simulink model "VFlexP"  (R2025a)
settings: Solver=ode23tb  StartTime=0.0  StopTime=40  FixedStep=5e-5
model workspace (MAT data in the model file):
  DCop_DCBUCK : object (value not decoded)
  Grid_CCVSC_idx = [2; 3; 4; 5; 6; 7; 8; 9; 10; 11; 12]
  Grid_CCVSCs = 1
  Grid_CCVSCs_buses = 1
  Grid_CCVSCs_toM = [0 1 0 0 0 0 0 0 0 0 0 0 ... (781 elements, 71x11)]
  Grid_C_Lines = [0.1 0.1 0.1 0.1]
  Grid_Cbuses = [0.05000002 0.10000002 0.10000002 0.10000002 0.05000002]
  Grid_DC : object (value not decoded)
  Grid_DCop_DCBUCK : object (value not decoded)
  Grid_DCop_DC_PES : object (value not decoded)
  Grid_DFIGs = 1
  Grid_DFIGs_buses = 1
  Grid_DGs : string (value not decoded)
  Grid_From_buses = [1 2 4 4]
  Grid_GFls = 1
  Grid_GFls_buses = 1
  Grid_GFr_idx = [1; 2; 3]
  Grid_GFrs = 1
  Grid_GFrs_buses = 1
  Grid_GFrs_toM = [1 0 0 0 0 0 0 0 0 1 0 0 ... (15 elements, 5x3)]
  Grid_IG_idx = 1
  Grid_IGs = 1
  Grid_IGs_buses = 1
  Grid_IGs_toM = [1; 0]
  Grid_L_Lines = [0.5 0.5 0.5 0.5]
  Grid_L_Loads = [0.000959999944704 0.000156249997559 0.00154855477548]
  Grid_Lines_fromM : object (value not decoded)
  Grid_Lines_toM : object (value not decoded)
  Grid_Load_buses = [2; 3; 4]
  Grid_Load_busesDC = []
  Grid_MGES_idx = [1; 2; 3]
  Grid_MGESs = 1
  Grid_MGESs_buses = [1; 5; 3]
  Grid_MGESs_toM = [1 0 0 0 0 0 0 0 0 1 0 0 ... (15 elements, 5x3)]
  Grid_MSGs = 1
  Grid_MSGs_buses = 1
  Grid_Nbuses = 5
  Grid_PQ_gen = [3; 2; 2]
  Grid_Ploads = [1250 4000 1250]
  Grid_PloadsDC = []
  Grid_Ps_lf = [0.274439537683 0.78 0.3]
  Grid_Qloads = [0.3 0.5 0.5]
  Grid_Qs_lf = [-0.0366071562958 0.126505596722 -0.0162964024532]
  Grid_R_Lines = [0.01 0.01 0.01 0.01]
  Grid_R_Loads = [3.9999997696 1.24999998047 3.8713869387]
  Grid_R_Loads_DC = 0
  Grid_Rcf = [50000000 50000000 50000000 50000000 50000000]
  Grid_SCs = 1
  Grid_SCs_buses = 1
  Grid_SG_idx = 1
  Grid_SGs = 1
  Grid_SGs_buses = 1
  Grid_SGs_toM = [1; 0]
  Grid_To_buses = [2 3 3 5]
  Grid_VCVSC_idx = [1; 2; 3; 4; 5; 6; 7; 8; 9; 10; 11; 12]
  Grid_VCVSCs = 1
  Grid_VCVSCs_buses = [1; 2; 3; 6; 8; 9; 12; 58; 59; 60; 63; 65]
  Grid_VCVSCs_toM = [1 0 0 0 0 0 0 0 0 0 0 0 ... (852 elements, 71x12)]
  Grid_VSM_idx = [1; 2; 3]
  Grid_VSMs = 1
  Grid_VSMs_buses = 1
  Grid_VSMs_toM = [1 0 0 0 0 0 0 0 0 1 0 0 ... (15 elements, 5x3)]
  Grid_admitt_matrix = [2.15353135314-19.7953135314i  -1.9801980198+19.801980198i; -1.9801980198+19.801980198i  2.15353135314-19.7953135314i]
  Grid_admitt_matrix_noloads = [1.98686468647-19.7953135314i  -1.9801980198+19.801980198i; -1.9801980198+19.801980198i  1.98686468647-19.7953135314i]
  Grid_bus = [1; 2; 6; 7; 8]
  Grid_busDC_complexity = [1 1 1]
  Grid_busDC_complexity_PF = [2 2 2]
  Grid_bus_complexity = [1 1 1 1 1]
  Grid_bus_complexity_PF = [1 1 1 1 1]
  Grid_buses_lf = [1; 5; 3]
  Grid_conductance_matrix = [100.00000002  -100  0; -100  200.00000002  -100; 0  -100  100.00000002]
  Grid_conductance_matrix_noloads = [100.00000002  -100  0; -100  200.00000002  -100; 0  -100  100.00000002]
  Grid_fref : object (value not decoded)
  Grid_gen_static_params : mBase (value not decoded)
  Grid_iPs_lf = [3.64378984326 1.28205128205 3.33333333333]
  Grid_iQs_lf = [-27.3170631425 7.90478860943 -61.3632366329]
  Grid_iadmitt_matrix = [2.88165849328-0.0982918688642i  2.87905051706-0.123273862303i; 2.87905051706-0.123273862303i  2.88165849328-0.0982918688642i]
  Grid_iadmitt_matrix_noloads = [37.5012524798-37.4874983544i  37.4987475202-37.5125016456i; 37.4987475202-37.5125016456i  37.5012524798-37.4874983544i]
  Grid_iconductance_matrix = [16666671.4556  16666671.4489  16666671.4456; 16666671.4489  16666671.4522  16666671.4489; 16666671.4456  16666671.4489  16666671.4556]
  Grid_iconductance_matrix_noloads = [16666671.4556  16666671.4489  16666671.4456; 16666671.4489  16666671.4522  16666671.4489; 16666671.4456  16666671.4489  16666671.4556]
  Grid_init_OK_bool = 1
  Grid_intconv_PF : object (value not decoded)
  Grid_lf_op : op_report (value not decoded)
  Grid_lineDC_complexity = [1 1]
  Grid_lineDC_complexity_PF = [2 2]
  Grid_line_complexity = [1 1 1 1]
  Grid_line_complexity_PF = [3 3 3 3]
  Grid_loadDC_complexity = []
  Grid_loadDC_complexity_PF = []
  Grid_load_complexity = [3 3 3]
  Grid_load_complexity_PF = [4 4 4]
  Grid_opDC_CCVSC : object (value not decoded)
  Grid_opDC_VSM : object (value not decoded)
  Grid_opGFr : object (value not decoded)
  Grid_opVCVSC : object (value not decoded)
  Grid_op_CCVSC : object (value not decoded)
  Grid_op_IG : object (value not decoded)
  Grid_op_MGES : object (value not decoded)
  Grid_op_SG : object (value not decoded)
  Grid_op_VSM : object (value not decoded)
  Grid_shift_lines = [0 0 0 0]
  Grid_tap_lines = [1 1 1 1]
  Grid_v_buses_mod = [1 1 1 0.9837920967 1]
  LinsysParamChangeStruct : Param1 (value not decoded)
  Lline = 0.01
  Rline = 1e-05
  linsys : object (value not decoded)
symbols that are objects in the model workspace (value not decoded): Grid_DCop_DC_PES, Grid_DCop_DCBUCK, Grid_op_CCVSC, Grid_op_IG, Grid_op_MGES, Grid_op_SG, Grid_op_VSM, Grid_opDC_CCVSC, Grid_opDC_VSM, Grid_opGFr, Grid_opVCVSC
undefined symbols (not defined in the file): block_buses_DC, block_idx, CCVSC_idx, Cf, costs, costs2, D, DFIGs_nodes, DiscIntNeverNeededParam, entity, Fb, Fi, From_nodes, grid_linsys, Grid_op_DFIG, Grid_op_DFIG_PQ, Grid_op_MSG, Grid_op_SC, Grid_op_VCVSC, H, initial_states_grid, K_1, K_3, K_5, K_A, K_C, K_IM, K_IR, K_P, K_PM, K_PR, K_S1, K_S2, K_S3, Ki_w, Kic, Kiv, Kp_id, Kp_theta, Kp_w, Kpc, Kpv, last_send, Lc, Lf, Lfd, Lkd1, Lkd2, Lkq1, Lkq2, Lkq3, Lmd, Lmq, Lsd, Lsq, m, M, Matrix_flux_to_i, mp, MSGs_buses ... (+44)
libraries: simulink x1048, eeGeneralControl x12
(part 6 of 50)

== system VFlexP/Grid/Generators/MGES ==
  note: Governor
  note: do not rename this block, conditions to initialise the generator from PF result are set on this block's output
  note: port number 1
  note: port number 2
  note: AVR
  elec_in : Inport
  v : Inport  Port=2
  AVR_Exciter : Subsystem  mask{T_s=T_e}
      mask prompts: T_s "Filter time constant"
  AVR_Vmeas_Filter : Subsystem  mask{T_r=T_v}
      mask prompts: T_r "Filter time constant"
  AVR_Vmeas_Filter1 : Subsystem  mask{T_r=0.01}
      mask prompts: T_r "Filter time constant"
  AVR_Vmeas_Filter2 : Subsystem  Commented=through  mask{T_r=0.01}
      mask prompts: T_r "Filter time constant"
      mask Display:
      | try
      |     dpoly(1, [T_r, 1])
      | catch
      | end
  AVR_Vmeas_Filter3 : Subsystem  mask{T_r=T_7p}
      mask prompts: T_r "Filter time constant"
  Abs : Abs  SaturateOnIntegerOverflow=off
  Assignment : Assignment  NumberOfDimensions=2  DiagnosticForDimensions=Warning  IndexOptions=Assign all,Index vector (dialog)  Indices=1,block_idx  OutputSizes=1,1
  Cast To Boolean : DataTypeConversion  OutDataTypeStr=boolean  SaturateOnIntegerOverflow=off  RndMeth=Floor
  Cast To Double : DataTypeConversion  OutDataTypeStr=double  SaturateOnIntegerOverflow=off  RndMeth=Floor
  Cast To Double1 : DataTypeConversion  OutDataTypeStr=double  SaturateOnIntegerOverflow=off  RndMeth=Floor
  Complex to Magnitude-Angle1 : ComplexToMagnitudeAngle  Output=Magnitude
  Complex to Magnitude-Angle2 : ComplexToMagnitudeAngle  Output=Magnitude
  Constant : Constant  Value=zeros(1, length(block_buses))  VectorParams1D=off
  Display : Display
  Divide : Product  Inputs=*/
  Electromagnetic : Subsystem  Variant=on  VariantControlMode=label  LabelModeActiveChoice=order 8
  For Each Subsystem : Subsystem  TreatAsAtomicUnit=on
  Gain : Gain  Gain=1./R_p
  Gain1 : Gain  Gain=K_5
  Gain10 : Gain  Gain=Ps_lf(block_idx)
  Gain11 : Gain  Gain=K_S2
  Gain12 : Gain  Gain=K_S3
  Gain13 : Gain  Gain=0.001
  Gain2 : Gain  Gain=-1
  Gain3 : Gain  Gain=gen_static_params.mBase(block_idx)'./Sb
  Gain4 : Gain  Gain=K_3
  Gain5 : Gain  Gain=K_1
  Gain6 : Gain  Gain=K_A
  Gain7 : Gain  Gain=gen_static_params.mBase(block_idx)'./Sb
  Gain8 : Gain  Gain=K_S1
  Gain9 : Gain  Gain=Sb./gen_static_params.mBase(block_idx)'
  Integrator1 : Integrator  InitialCondition=Grid_op_MGES.op.States(13).x'
  Integrator2 : Integrator  InitialCondition=Grid_op_MGES.op.States(14).x'
  Integrator3 : Integrator  InitialCondition=Grid_op_MGES.op.States(15).x'
  LPF1 : Subsystem  mask{T_s=T_6}
      mask prompts: T_s "Filter time constant"
  LPF2 : Subsystem  mask{T_s=T_3}
      mask prompts: T_s "Filter time constant"
  LPF3 : Subsystem  mask{T_s=T_4}
      mask prompts: T_s "Filter time constant"
  LPF4 : Subsystem  Commented=through  mask{T_s=0.01}
      mask prompts: T_s "Filter time constant"
      mask Display:
      | try
      |     dpoly(1, [T_s, 1])
      | catch
      | end
  LPF5 : Subsystem  Commented=through  mask{T_s=0.01}
      mask prompts: T_s "Filter time constant"
      mask Display:
      | try
      |     dpoly(1, [T_s, 1])
      | catch
      | end
  LPF6 : Subsystem  mask{T_s=T_5}
      mask prompts: T_s "Filter time constant"
  LeadLag : Subsystem
  LeadLag1 : Subsystem  mask{T_2=T_1p, T_1=T_2p}
      mask help:
      | Transfer function:
      |
      |   1 + sT_2
      | ---------------
      |   1 + sT_1
  LeadLag2 : Subsystem  mask{T_2=T_3p, T_1=T_4p}
      mask help:
      | Transfer function:
      |
      |   1 + sT_2
      | ---------------
      |   1 + sT_1
  Matrix Concatenate : Concatenate  NumInputs=6  Mode=Multidimensional array
  Matrix Concatenate1 : Concatenate  NumInputs=3  Mode=Multidimensional array
  Memory : Memory  InitialCondition=1
  Memory1 : Memory  InitialCondition=1
  Memory2 : Memory  InitialCondition=1
  PI1 : Subsystem
  PI2 : Subsystem
  Product{,1..5} (6 alike) : Product
  Real-Imag to Complex : RealImagToComplex
  Real-Imag to Complex1 : RealImagToComplex
  Real-Imag to Complex2 : RealImagToComplex
  Reference frame transform1 : Subsystem
  Reference frame transform3 : Subsystem
  Rotor axis : Subsystem
  Scope : Scope
      settings: ActiveDisplayYMinimum=-1  ActiveDisplayYMaximum=1  DataLoggingVariableName=ScopeData13
  Scope1 : Scope
      settings: ActiveDisplayYMinimum=-0.058141408811601208  ActiveDisplayYMaximum=2.1702525958532117  DataLoggingVariableName=ScopeData3
  Scope2 : Scope
      settings: ActiveDisplayYMinimum=-0.402690614368146  ActiveDisplayYMaximum=1.3038964261892889  DataLoggingVariableName=ScopeData9
  Scope3 : Scope  NumInputPorts=2
      settings: ActiveDisplayYMinimum=0.29123  ActiveDisplayYMaximum=1.9416  DataLoggingVariableName=ScopeData3
  Selector : Selector  NumberOfDimensions=2  InputPortWidth=3  IndexOptions=Index vector (dialog),Index vector (dialog)  Indices=1,block_idx  OutputSizes=1,1
  Selector1 : Selector  NumberOfDimensions=2  InputPortWidth=3  IndexOptions=Index vector (dialog),Index vector (dialog)  Indices=2,block_idx  OutputSizes=1,1
  Selector2 : Selector  NumberOfDimensions=2  InputPortWidth=3  IndexOptions=Index vector (dialog),Index vector (dialog)  Indices=3,block_idx  OutputSizes=1,1
  Selector3 : Selector  NumberOfDimensions=2  InputPortWidth=3  IndexOptions=Index vector (dialog),Index vector (dialog)  Indices=4,block_idx  OutputSizes=1,1
  Selector4 : Selector  NumberOfDimensions=2  InputPortWidth=3  IndexOptions=Index vector (dialog),Index vector (dialog)  Indices=5,block_idx  OutputSizes=1,1
  Selector5 : Selector  NumberOfDimensions=2  InputPortWidth=3  IndexOptions=Index vector (dialog),Index vector (dialog)  Indices=1,block_buses  OutputSizes=1,1
  Selector6 : Selector  NumberOfDimensions=2  InputPortWidth=3  IndexOptions=Index vector (dialog),Index vector (dialog)  Indices=2,block_buses  OutputSizes=1,1
  Selector7 : Selector  InputPortWidth=length(fref.ref_units)  IndexOptions=Index vector (dialog)  Indices=block_fref  OutputSizes=1
  Selector8 : Selector  InputPortWidth=length(fref.ref_units)  IndexOptions=Index vector (dialog)  Indices=block_fref  OutputSizes=1
  Signal Specification : SignalSpecification  Dimensions=[6 length(buses_lf)]
  Signal Specification1 : SignalSpecification  Dimensions=[3 length(block_buses)]
  Subsystem : Subsystem
  Subsystem1 : Subsystem
  Subsystem4 : Subsystem  Commented=through  mask{T_2=T_2, T_1=T_1}
      mask help:
      | Transfer function:
      |
      |   1 + sT_2
      | ---------------
      |   1 + sT_1
  Sum{,3,5..6,8} (5 alike) : Sum  Inputs=|++
  Sum1 : Sum  Inputs=|-+
  Sum10 : Sum  Inputs=+|+|-
  Sum2 : Sum  Inputs=|+-
  Sum4 : Sum  Inputs=|-+
  Sum7 : Sum  Inputs=|+-
  Terminator{2..5} (4 alike) : Terminator
  Torque : Subsystem
      settings: PortSchema="{\"entries\":[{\"content\":{\"sides\":[{\"content\":{\"connectorIds\":[\"In1\"]},\"type\":\"ConnectorPlacement.EquallySpacedRectSide\",\"uuid\":\"b7abd3bc-22dd-4669-aa40-98bc76884565\"},{\"content\":{\"connectorIds\":[\"In2\",\"In3\",\"Out1\"],\"side\":\"RIGHT\"},\"type\":\"ConnectorPlacement.EquallySpacedRectSide\",\"uuid\":\"e9abb552-b46d-48ed-aa1f-0e9dac604fea\"},{\"content\":{\"connectorIds\":[],\"side\":\"TOP\"},\"type\":\"ConnectorPlacement.EquallySpacedRectSide\",\"uuid\":\"4b14997d-8f32-4cfb-8a1b-18cffb093d28\"}]},\"type\":\"ConnectorPlacement.EquallySpacedConnector\",\"uuid\":\"d6624493-e930-4f0d-8cbe-17f96cb72edc\"}],\"packageUris\":[\"http://schema.mathworks.com/mf0/Connector/R2020b\"],\"version\":\"1.0\"}"
  WOF_d : Subsystem
  WOF_d1 : Subsystem
  Zero1 : Constant  Value=zeros(6, length(buses_lf))  VectorParams1D=off  OutDataTypeStr=Inherit: Inherit via back propagation
  connect : Subsystem
  theta : Integrator  InitialCondition=Grid_op_MGES.op.States(33).x'  UpperSaturationLimit=2*pi  LowerSaturationLimit=0
  trim_output : Subsystem
  elec_out : Outport
  i : Outport  Port=2
  wires:
  LPF5/1(out) -> [Q_s]
  Reference frame transform1/2(out_q) -> Gain7/1
  Product/1 -> Sum4/1
  Product1/1 -> Sum4/2
  theta/1 -> [theta]
  Gain2/1 -> Reference frame transform1/2(theta)
  [theta] -> Reference frame transform3/2(theta)
  LPF6/1(out) -> Gain4/1, LPF1/1(in)
  [theta] -> Gain2/1
  LPF2/1(out) -> LPF3/1(in)
  Sum4/1 -> LPF5/1(in)
  Sum5/1 -> LPF4/1(in)
  Product3/1 -> Sum5/2
  [omega_ref] -> Selector7/1  "ref_omega"
  Product2/1 -> Sum5/1
  Reference frame transform1/1(out_d) -> Gain3/1
  Subsystem4/1(Out1) -> LPF2/1(in)
  LPF4/1(out) -> [P_s]
  [P_s] -> Matrix Concatenate/2  "P_s"
  [omega] -> Matrix Concatenate/1  "omega"
  Complex to Magnitude-Angle1/1 -> AVR_Vmeas_Filter2/1(in)  "v"
  [Q_s] -> Matrix Concatenate/4  "Q_s"
  Selector3/1 -> [Q_s_to_follow_own]
  Selector/1 -> [omega_to_follow_own]
  Selector1/1 -> Gain10/1
  Selector2/1 -> [v_to_follow_own]
  [connect] -> Memory1/1
  [connected] -> Memory/1
  Cast To Double1/1 -> Matrix Concatenate/5
  Cast To Double/1 -> Matrix Concatenate/6
  Real-Imag to Complex1/1 -> Complex to Magnitude-Angle1/1
  [vdout] -> Product/1, Product2/1
  [vqout] -> Product3/1, Product1/2
  [v_d_PCC] -> Real-Imag to Complex1/1  "vod"
  [v_q_PCC] -> Real-Imag to Complex1/2  "voq"
  connect/3(connected) -> [connected]
  [connect] -> connect/3(connect)
  connect/1(id_real) -> Real-Imag to Complex2/1, trim_output/1(id), Matrix Concatenate1/1, Product1/1, Product2/2
  Selector4/1 -> Cast To Boolean/1
  Cast To Boolean/1 -> Memory2/1
  Zero1/1 -> Assignment/1
  Signal Specification/1 -> elec_out/1
  elec_in/1 -> Selector4/1, Selector3/1, Selector2/1, Selector1/1, Selector/1
  Assignment/1 -> Signal Specification/1
  Matrix Concatenate/1 -> Assignment/2
  Matrix Concatenate1/1 -> Signal Specification1/1
  Signal Specification1/1 -> For Each Subsystem/1(In1)
  Constant/1 -> Matrix Concatenate1/3
  For Each Subsystem/1(Out1) -> i/1
  connect/2(iq_real) -> Product3/2, Product/2, Real-Imag to Complex2/2, trim_output/2(iq), Matrix Concatenate1/2
  trim_output/3(Out3) -> Terminator4/1
  trim_output/1(Out1) -> Terminator2/1
  trim_output/4(Out4) -> Terminator5/1
  trim_output/2(Out2) -> Terminator3/1
  v/1 -> Selector6/1, Selector5/1
  Selector5/1 -> [vdout], trim_output/3(vd)
  Selector6/1 -> [vqout], trim_output/4(vq)
  [vqout] -> Reference frame transform3/3(in_q)
  [vdout] -> Reference frame transform3/1(in_d)
  Reference frame transform3/1(out_d) -> [v_d_PCC]
  Reference frame transform3/2(out_q) -> [v_q_PCC]
  Memory/1 -> Cast To Double/1
  Gain10/1 -> [P_s_to_follow_own]
  Memory1/1 -> Cast To Double1/1
  Memory2/1 -> [connect]
  Selector7/1 -> Sum1/2
  Selector8/1 -> Product4/2
  [omega_base] -> Selector8/1
  Product4/1 -> theta/1
  Sum1/1 -> Product4/1
  Gain/1 -> Subsystem4/1(In1)
  Sum2/1 -> Gain/1
  Integrator1/1 -> Sum10/2
  Gain6/1 -> PI2/1(In1)
  AVR_Vmeas_Filter/1(out) -> Sum10/3, Subsystem1/1(vt)
  LeadLag/1(Out1) -> AVR_Exciter/1(in)
  [v_d_PCC] -> Real-Imag to Complex/1
  Abs/1 -> AVR_Vmeas_Filter/1(in)  "v"
  [v_q_PCC] -> Real-Imag to Complex/2
  Real-Imag to Complex/1 -> Abs/1
  AVR_Vmeas_Filter1/1(out) -> Sum2/2
  AVR_Vmeas_Filter2/1(out) -> Matrix Concatenate/3, Scope3/1
  Real-Imag to Complex2/1 -> Complex to Magnitude-Angle2/1
  Complex to Magnitude-Angle2/1 -> Scope3/2  "v"
  Electromagnetic/2(isq) -> [isq], Torque/3(isq), Reference frame transform1/3(in_q)
  Electromagnetic/1(isd) -> Scope2/1, Reference frame transform1/1(in_d), Torque/2(isd), [isd]
  [v_d_PCC] -> Electromagnetic/1(vsd)
  [v_q_PCC] -> Electromagnetic/2(vsq)
  Electromagnetic/3(psi) -> Torque/1(psi)
  Divide/1 -> Display/1, Rotor axis/2(tm)
  Electromagnetic/4(ifd) -> [ifd]
  PI2/1(Out1) -> LeadLag/1(In1)
  AVR_Exciter/1(out) -> PI1/1(In1)
  [ifd] -> Subsystem1/2(ifd)
  PI1/1(vfd) -> Product5/1
  Subsystem1/1(V_B) -> Product5/2
  LPF3/1(out) -> Gain5/1, LPF6/1(in)
  LPF1/1(out) -> Gain1/1
  Gain1/1 -> Sum/2
  Rotor axis/1(wr) -> Electromagnetic/4(ws), [omega], Scope1/1, Sum1/1, Divide/2, AVR_Vmeas_Filter1/1(in)
  Sum3/1 -> Sum/1
  Gain4/1 -> Sum3/2
  Gain5/1 -> Sum3/1
  Gain3/1 -> connect/1(id)
  Gain7/1 -> connect/2(iq)
  WOF_d/1(Out1) -> WOF_d1/1(In1)
  Gain8/1 -> LeadLag1/1(In1)
  LeadLag1/1(Out1) -> LeadLag2/1(In1)
  [omega] -> WOF_d/1(In1)
  WOF_d1/1(Out1) -> Sum6/1
  Sum6/1 -> Subsystem/1(in)
  Subsystem/1(out) -> Sum7/1
  Sum7/1 -> Gain8/1
  Gain12/1 -> Sum6/2
  Gain11/1 -> Sum7/2, Gain12/1
  AVR_Vmeas_Filter3/1(out) -> Gain11/1
  [P_s] -> Gain9/1
  Integrator2/1 -> Sum2/1
  Torque/1(te) -> Rotor axis/1(te)
  Sum10/1 -> Gain13/1
  Gain13/1 -> Gain6/1
  Product5/1 -> Electromagnetic/3(vfd)
  Sum/1 -> Sum8/1
  Sum8/1 -> Divide/1
  Integrator3/1 -> Sum8/2
  Gain9/1 -> AVR_Vmeas_Filter3/1(in)
  LeadLag2/1(Out1) -> Sum10/1

== system VFlexP/Grid/Generators/MSG ==
  note: port number 1
  note: port number 2
  elec_in : Inport
  v : Inport  Port=2
  Assignment : Assignment  NumberOfDimensions=2  DiagnosticForDimensions=Warning  IndexOptions=Assign all,Index vector (dialog)  Indices=1,block_idx  OutputSizes=1,1
  Cast To Boolean : DataTypeConversion  OutDataTypeStr=boolean  SaturateOnIntegerOverflow=off  RndMeth=Floor
  Cast To Double : DataTypeConversion  OutDataTypeStr=double  SaturateOnIntegerOverflow=off  RndMeth=Floor
  Cast To Double1 : DataTypeConversion  OutDataTypeStr=double  SaturateOnIntegerOverflow=off  RndMeth=Floor
  Complex to Magnitude-Angle1 : ComplexToMagnitudeAngle  Output=Magnitude
  Constant : Constant
  Constant1 : Constant  Value=1.028
  Constant2 : Constant  Value=zeros(1, length(block_buses))  VectorParams1D=off
  Constant6 : Constant  Value=0
  Constant7 : Constant  Value=0.022
  Display : Display
  For Each Subsystem : Subsystem  TreatAsAtomicUnit=on
  GRID CONVERTER CONTROL : Subsystem
  Gain : Gain  Gain=-1
  Gain1 : Gain  Gain=-1
  Gain3 : Gain  Gain=Ps_lf(block_idx)
  Gain4 : Gain  Gain=-1
  Gain5 : Gain
  Gain9 : Gain  Gain=1./Ps_lf(block_idx)
  MACHINE CONVERTER CONTROL : Subsystem
  Matrix Concatenate : Concatenate  NumInputs=6  Mode=Multidimensional array
  Matrix Concatenate1 : Concatenate  NumInputs=3  Mode=Multidimensional array
  Memory : Memory  InitialCondition=1
  Product{,1,3,5..6} (5 alike) : Product
  Real-Imag to Complex3 : RealImagToComplex
  Reference frame transform3 : Subsystem
  Reference frame transform5 : Subsystem
  Rotor axis : Subsystem
  Scope : Scope
      settings: ActiveDisplayYMinimum=1.0278  ActiveDisplayYMaximum=1.0294
  Scope1 : Scope
      settings: ActiveDisplayYMinimum=-1.2398  ActiveDisplayYMaximum=-0.95917  DataLoggingVariableName=ScopeData3
  Selector : Selector  NumberOfDimensions=2  InputPortWidth=3  IndexOptions=Index vector (dialog),Index vector (dialog)  Indices=1,block_idx  OutputSizes=1,1
  Selector2 : Selector  InputPortWidth=length(fref.ref_units)  IndexOptions=Index vector (dialog)  Indices=block_fref  OutputSizes=1
  Selector3 : Selector  NumberOfDimensions=2  InputPortWidth=3  IndexOptions=Index vector (dialog),Index vector (dialog)  Indices=2,block_idx  OutputSizes=1,1
  Selector4 : Selector  NumberOfDimensions=2  InputPortWidth=3  IndexOptions=Index vector (dialog),Index vector (dialog)  Indices=3,block_idx  OutputSizes=1,1
  Selector5 : Selector  NumberOfDimensions=2  InputPortWidth=3  IndexOptions=Index vector (dialog),Index vector (dialog)  Indices=4,block_idx  OutputSizes=1,1
  Selector6 : Selector  NumberOfDimensions=2  InputPortWidth=3  IndexOptions=Index vector (dialog),Index vector (dialog)  Indices=5,block_idx  OutputSizes=1,1
  Selector7 : Selector  NumberOfDimensions=2  InputPortWidth=3  IndexOptions=Index vector (dialog),Index vector (dialog)  Indices=1,block_buses  OutputSizes=1,1
  Selector8 : Selector  NumberOfDimensions=2  InputPortWidth=3  IndexOptions=Index vector (dialog),Index vector (dialog)  Indices=2,block_buses  OutputSizes=1,1
  Signal Specification : SignalSpecification  Dimensions=[6 length(buses_lf)]
  Signal Specification1 : SignalSpecification  Dimensions=[3 length(block_buses)]
  Stator circuit MSG : Subsystem
  Step : Step  Before=1  After=1.1  SampleTime=0
  Subsystem : Subsystem
  Sum4 : Sum  Inputs=|++
  Sum5 : Sum  Inputs=|-+
  Terminator{,5..8} (5 alike) : Terminator
  Torque : Subsystem
      settings: PortSchema="{\"entries\":[{\"content\":{\"sides\":[{\"content\":{\"connectorIds\":[\"In1\"]},\"type\":\"ConnectorPlacement.EquallySpacedRectSide\",\"uuid\":\"b7abd3bc-22dd-4669-aa40-98bc76884565\"},{\"content\":{\"connectorIds\":[\"In2\",\"In3\"],\"side\":\"RIGHT\"},\"type\":\"ConnectorPlacement.EquallySpacedRectSide\",\"uuid\":\"e9abb552-b46d-48ed-aa1f-0e9dac604fea\"},{\"content\":{\"connectorIds\":[],\"side\":\"TOP\"},\"type\":\"ConnectorPlacement.EquallySpacedRectSide\",\"uuid\":\"4b14997d-8f32-4cfb-8a1b-18cffb093d28\"},{\"content\":{\"connectorIds\":[\"Out1\"],\"side\":\"BOTTOM\"},\"type\":\"ConnectorPlacement.EquallySpacedRectSide\",\"uuid\":\"0ad577f8-eb9c-4d21-85f4-8d3c6640245c\"}]},\"type\":\"ConnectorPlacement.EquallySpacedConnector\",\"uuid\":\"d6624493-e930-4f0d-8cbe-17f96cb72edc\"}],\"packageUris\":[\"http://schema.mathworks.com/mf0/Connector/R2020b\"],\"version\":\"1.0\"}"
  Vc control : Subsystem
  Zero : Constant  Value=0  OutDataTypeStr=Inherit: Inherit via back propagation
  Zero1 : Constant  Value=zeros(6, length(buses_lf))  VectorParams1D=off  OutDataTypeStr=Inherit: Inherit via back propagation
  Zero2 : Constant  Value=0  OutDataTypeStr=Inherit: Inherit via back propagation
  connect : Subsystem
  iaq_ref : Integrator  InitialCondition=Grid_op_MSG.op.States(14).x'
  psi->i : Subsystem
  tm : Integrator  InitialCondition=Grid_op_MSG.op.States(15).x'
  trim_output : Subsystem
  elec_out : Outport
  i : Outport  Port=2
  wires:
  Product5/1 -> Sum5/1
  [v_d_PCC] -> Product1/1, Product5/1  "vod"
  Product3/1 -> Sum4/2
  [id_out] -> Product1/2, Product6/2  "iod"
  Sum5/1 -> [Q_s]
  [v_q_PCC] -> Product6/1, Product3/1  "voq"
  Product6/1 -> Sum5/2
  Sum4/1 -> [P_s]
  Product1/1 -> Sum4/1
  [iq_out] -> Product3/2, Product5/2  "ioq"
  Signal Specification/1 -> elec_out/1
  Gain4/1 -> Reference frame transform3/2(theta)
  For Each Subsystem/1(Out1) -> i/1
  [omega_ref] -> Selector2/1
  trim_output/2(Out2) -> Terminator6/1
  Selector5/1 -> [Q_s_to_follow_own]
  [iad] -> GRID CONVERTER CONTROL/3(iad)
  Vc control/1(iad_ref) -> [iad_ref]
  [vsd] -> Vc control/2(vsd)
  [vad] -> Vc control/6(vad)
  [te] -> Rotor axis/1(te)
  [omega_ref] -> Terminator/1  "ref_omega"
  Assignment/1 -> Signal Specification/1
  GRID CONVERTER CONTROL/1(vad) -> [vad]
  [iaq] -> Vc control/9(iaq)
  GRID CONVERTER CONTROL/2(vaq) -> [vaq]
  [vsq] -> Vc control/3(vsq)
  psi->i/3(isq) -> [isq]
  [iad_ref] -> GRID CONVERTER CONTROL/2(iad_ref)
  Constant/1 -> Vc control/1(Vc_2_ref)
  iaq_ref/1 -> GRID CONVERTER CONTROL/4(iaq_ref)
  [iad] -> Vc control/8(iad)
  [vdout] -> Reference frame transform3/1(in_d)
  Zero/1 -> Gain4/1
  Gain9/1 -> Matrix Concatenate/2
  [P_s] -> Gain9/1  "P_s"
  Matrix Concatenate1/1 -> Signal Specification1/1
  trim_output/4(Out4) -> Terminator8/1
  Selector8/1 -> [vqout], trim_output/4(vq)
  Constant2/1 -> Matrix Concatenate1/3
  trim_output/3(Out3) -> Terminator7/1
  Cast To Boolean/1 -> [connect]
  v/1 -> Selector8/1, Selector7/1
  Signal Specification1/1 -> For Each Subsystem/1(In1)
  [vd] -> GRID CONVERTER CONTROL/1(vd)
  [ws] -> GRID CONVERTER CONTROL/6(ws)
  Selector7/1 -> trim_output/3(vd), [vdout]
  Gain5/1 -> Reference frame transform5/2(theta)
  elec_in/1 -> Selector6/1, Selector5/1, Selector4/1, Selector3/1, Selector/1
  connect/2(iq_real) -> trim_output/2(iq), Matrix Concatenate1/2
  [connect] -> Cast To Double1/1
  Cast To Double/1 -> Matrix Concatenate/6
  Cast To Double1/1 -> Matrix Concatenate/5
  Selector6/1 -> Cast To Boolean/1
  [Q_s] -> Matrix Concatenate/4  "Q_s"
  connect/1(id_real) -> trim_output/1(id), Matrix Concatenate1/1
  psi->i/2(i) -> Stator circuit MSG/3(i), Scope1/1, [i]
  trim_output/1(Out1) -> Terminator5/1
  [ws] -> Matrix Concatenate/1  "omega"
  Zero1/1 -> Assignment/1
  Selector/1 -> [omega_to_follow_own]
  Selector3/1 -> Gain3/1
  Selector4/1 -> [v_to_follow_own]
  Gain3/1 -> [P_s_to_follow_own]
  [vaq] -> Vc control/7(vaq)
  [isd] -> Vc control/4(isd)
  Matrix Concatenate/1 -> Assignment/2
  [iaq] -> GRID CONVERTER CONTROL/5(iaq)
  Zero2/1 -> Gain5/1
  psi->i/1(isd) -> [isd]
  [connect] -> connect/3(connect)
  [iad] -> Gain/1
  [connected] -> Memory/1
  [isq] -> Vc control/5(isq)
  connect/3(connected) -> [connected]
  Memory/1 -> Cast To Double/1
  Stator circuit MSG/1(psi) -> Torque/1(psi), psi->i/1(psi), Display/1
  Rotor axis/1(wr) -> Scope/1, [wr]
  Constant6/1 -> MACHINE CONVERTER CONTROL/1(isd_ref)
  [isq_ref] -> MACHINE CONVERTER CONTROL/3(isq_ref)
  MACHINE CONVERTER CONTROL/1(vsd) -> [vsd]
  [wr] -> MACHINE CONVERTER CONTROL/5(wr)
  MACHINE CONVERTER CONTROL/2(vsq) -> [vsq]
  Constant1/1 -> Subsystem/1(wref)
  [wr] -> Subsystem/2(wr)
  [ifd] -> MACHINE CONVERTER CONTROL/6(ifd)
  [vsd] -> Stator circuit MSG/1(vsd)
  [vsq] -> Stator circuit MSG/2(vsq)
  [vad] -> Stator circuit MSG/6(vad)
  [vaq] -> Stator circuit MSG/7(vaq)
  [ws] -> Stator circuit MSG/4(ws)
  [isd] -> Torque/2(isd)
  [isq] -> Torque/3(isq)
  Torque/1(te) -> [te]
  [vd] -> Stator circuit MSG/8(vd)
  [vq] -> Stator circuit MSG/9(vq)
  [wr] -> Stator circuit MSG/10(wr)
  [iaq] -> Gain1/1
  [v_q_PCC] -> Real-Imag to Complex3/2
  Real-Imag to Complex3/1 -> Complex to Magnitude-Angle1/1
  Complex to Magnitude-Angle1/1 -> Matrix Concatenate/3  "v"
  [v_d_PCC] -> Real-Imag to Complex3/1
  psi->i/5(iad) -> [iad]
  psi->i/6(iaq) -> [iaq]
  [vqout] -> Reference frame transform3/3(in_q)
  psi->i/4(ifd) -> [ifd]
  Constant7/1 -> Stator circuit MSG/5(vfd)
  Reference frame transform3/1(out_d) -> [vd]
  [vd] -> [v_d_PCC]
  Reference frame transform3/2(out_q) -> [vq]
  [vq] -> [v_q_PCC]
  Gain/1 -> Reference frame transform5/1(in_d)
  Gain1/1 -> Reference frame transform5/3(in_q)
  Reference frame transform5/1(out_d) -> [id_out], connect/1(id)
  Reference frame transform5/2(out_q) -> [iq_out], connect/2(iq)
  Subsystem/1(isq_ref) -> [isq_ref]
  [isd] -> MACHINE CONVERTER CONTROL/2(isd)
  [isq] -> MACHINE CONVERTER CONTROL/4(isq)
  tm/1 -> Product/1
  Step/1 -> Product/2
  Product/1 -> Rotor axis/2(tm)
  Selector2/1 -> [ws]

== system VFlexP/Grid/Generators/SC ==
  note: AVR
  note: do not rename this block, conditions to initialise the generator from PF result are set on this block's output
  note: port number 1
  note: port number 2
  elec_in : Inport
  v : Inport  Port=2
  AVR_Exciter : Subsystem  mask{T_s=T_e}
      mask prompts: T_s "Filter time constant"
      mask Display:
      | try
      |     dpoly(1, [T_s, 1])
      | catch
      | end
  AVR_LeadLag : Subsystem  mask{T_2=T_2, T_1=T_1}
      mask help:
      | Transfer function:
      |
      |   1 + sT_2
      | ---------------
      |   1 + sT_1
      mask Display:
      | try
      |     dpoly([T_2, 1], [T_1, 1])
      | catch
      | end
  AVR_MainRegulator : Subsystem  mask{T_s=T_A}
      mask prompts: T_s "Filter time constant"
      mask Display:
      | try
      |     dpoly(1, [T_s, 1])
      | catch
      | end
  AVR_Vmeas_Filter : Subsystem  mask{T_r=0.01}
      mask prompts: T_r "Filter time constant"
      mask Display:
      | try
      |     dpoly(1, [T_r, 1])
      | catch
      | end
  Abs : Abs  SaturateOnIntegerOverflow=off
  Assignment : Assignment  NumberOfDimensions=2  DiagnosticForDimensions=Warning  IndexOptions=Assign all,Index vector (dialog)  Indices=1,block_idx  OutputSizes=1,1
  Cast To Boolean : DataTypeConversion  OutDataTypeStr=boolean  SaturateOnIntegerOverflow=off  RndMeth=Floor
  Cast To Double : DataTypeConversion  OutDataTypeStr=double  SaturateOnIntegerOverflow=off  RndMeth=Floor
  Cast To Double1 : DataTypeConversion  OutDataTypeStr=double  SaturateOnIntegerOverflow=off  RndMeth=Floor
  Constant : Constant  Value=zeros(1, length(block_buses))  VectorParams1D=off
  For Each Subsystem : Subsystem  TreatAsAtomicUnit=on
  Gain1 : Gain  Gain=0.01
  Gain2 : Gain  Gain=-1
  Gain4 : Gain  Gain=3.4e-4
  Gain7 : Gain  Gain=0.001
  Gain8 : Gain  Gain=K_A
  Gain9 : Gain
  Integrator1 : Integrator  InitialCondition=Grid_op_SC.op.States(5).x'
  Integrator2 : Integrator  InitialCondition=Grid_op_SC.op.States(6).x'
  Integrator3 : Integrator  InitialCondition=Grid_op_SC.op.States(7).x'
  Matrix Concatenate : Concatenate  NumInputs=6  Mode=Multidimensional array
  Matrix Concatenate1 : Concatenate  NumInputs=3  Mode=Multidimensional array
  Memory : Memory  InitialCondition=1
  Memory1 : Memory  InitialCondition=1
  Memory2 : Memory  InitialCondition=1
  Product{,1..4} (5 alike) : Product
  Real-Imag to Complex : RealImagToComplex
  Reference frame transform1 : Subsystem
  Reference frame transform2 : Subsystem
  Rotor axis : Subsystem
  Selector : Selector  NumberOfDimensions=2  InputPortWidth=3  IndexOptions=Index vector (dialog),Index vector (dialog)  Indices=1,block_idx  OutputSizes=1,1
  Selector1 : Selector  NumberOfDimensions=2  InputPortWidth=3  IndexOptions=Index vector (dialog),Index vector (dialog)  Indices=2,block_idx  OutputSizes=1,1
  Selector2 : Selector  NumberOfDimensions=2  InputPortWidth=3  IndexOptions=Index vector (dialog),Index vector (dialog)  Indices=3,block_idx  OutputSizes=1,1
  Selector3 : Selector  NumberOfDimensions=2  InputPortWidth=3  IndexOptions=Index vector (dialog),Index vector (dialog)  Indices=4,block_idx  OutputSizes=1,1
  Selector4 : Selector  NumberOfDimensions=2  InputPortWidth=3  IndexOptions=Index vector (dialog),Index vector (dialog)  Indices=5,block_idx  OutputSizes=1,1
  Selector5 : Selector  NumberOfDimensions=2  InputPortWidth=3  IndexOptions=Index vector (dialog),Index vector (dialog)  Indices=1,block_buses  OutputSizes=1,1
  Selector6 : Selector  NumberOfDimensions=2  InputPortWidth=3  IndexOptions=Index vector (dialog),Index vector (dialog)  Indices=2,block_buses  OutputSizes=1,1
  Selector7 : Selector  InputPortWidth=length(fref.ref_units)  IndexOptions=Index vector (dialog)  Indices=block_fref  OutputSizes=1
  Selector8 : Selector  InputPortWidth=length(fref.ref_units)  IndexOptions=Index vector (dialog)  Indices=block_fref  OutputSizes=1
  Signal Specification : SignalSpecification  Dimensions=[6 length(buses_lf)]
  Signal Specification1 : SignalSpecification  Dimensions=[3 length(block_buses)]
  Stator circuit : Subsystem
  Sum1 : Sum  Inputs=|-+
  Sum2 : Sum  Inputs=|+-
  Sum4 : Sum  Inputs=|-+
  Sum5 : Sum  Inputs=|++
  Sum8 : Sum  Inputs=|-+
  Sum9 : Sum  Inputs=|++
  Terminator{2..5} (4 alike) : Terminator
  Torque : Subsystem
      settings: PortSchema="{\"entries\":[{\"content\":{\"sides\":[{\"content\":{\"connectorIds\":[\"In1\"]},\"type\":\"ConnectorPlacement.EquallySpacedRectSide\",\"uuid\":\"b7abd3bc-22dd-4669-aa40-98bc76884565\"},{\"content\":{\"connectorIds\":[\"In2\",\"In3\",\"Out1\"],\"side\":\"RIGHT\"},\"type\":\"ConnectorPlacement.EquallySpacedRectSide\",\"uuid\":\"e9abb552-b46d-48ed-aa1f-0e9dac604fea\"},{\"content\":{\"connectorIds\":[],\"side\":\"TOP\"},\"type\":\"ConnectorPlacement.EquallySpacedRectSide\",\"uuid\":\"4b14997d-8f32-4cfb-8a1b-18cffb093d28\"}]},\"type\":\"ConnectorPlacement.EquallySpacedConnector\",\"uuid\":\"d6624493-e930-4f0d-8cbe-17f96cb72edc\"}],\"packageUris\":[\"http://schema.mathworks.com/mf0/Connector/R2020b\"],\"version\":\"1.0\"}"
  Transport Delay : TransportDelay  DelayTime=0.0001  TransDelayFeedthrough=on
  Zero1 : Constant  Value=zeros(6, length(buses_lf))  VectorParams1D=off  OutDataTypeStr=Inherit: Inherit via back propagation
  connect : Subsystem
  psi->i : Subsystem
  theta : Integrator  InitialCondition=Grid_op_SC.op.States(17).x'  UpperSaturationLimit=2*pi  LowerSaturationLimit=0
  trim_output : Subsystem
  elec_out : Outport
  i : Outport  Port=2
  wires:
  Sum4/1 -> [Qe]
  Sum5/1 -> [Pe]
  [v_q_PCC] -> Real-Imag to Complex/2
  Real-Imag to Complex/1 -> Abs/1
  [v_d_PCC] -> Real-Imag to Complex/1
  [vqout] -> Product3/1, Product1/2
  [iq] -> Product3/2, Product/2
  Product/1 -> Sum4/1
  Product1/1 -> Sum4/2
  theta/1 -> [theta]
  psi->i/1(isd) -> Reference frame transform1/1(in_d), Torque/2(isd), [isd]
  psi->i/3(isq) -> [isq], Torque/3(isq), Reference frame transform1/3(in_q)
  Stator circuit/1(psi) -> Torque/1(psi), psi->i/1(psi)
  [v_q_PCC] -> Stator circuit/2(vsq)
  Gain2/1 -> Reference frame transform1/2(theta)
  Rotor axis/1(wr) -> Stator circuit/4(ws), Sum1/1, [omega]
  Torque/1(te) -> Rotor axis/1(te)
  [theta] -> Gain2/1
  psi->i/2(i) -> Stator circuit/3(i)
  [vdout] -> Product/1, Product2/1
  Product3/1 -> Sum5/2
  [omega_ref] -> Selector7/1  "ref_omega"
  Product2/1 -> Sum5/1
  [id] -> Product2/2, Product1/1
  [v_d_PCC] -> Stator circuit/1(vsd)
  Integrator2/1 -> Rotor axis/2(tm)
  Gain9/1 -> AVR_Exciter/1(in)
  AVR_Exciter/1(out) -> Gain4/1
  Sum2/1 -> Gain8/1
  AVR_LeadLag/1(Out1) -> Gain9/1
  Gain8/1 -> AVR_MainRegulator/1(in)
  AVR_MainRegulator/1(out) -> AVR_LeadLag/1(In1)
  Selector3/1 -> [Q_s_to_follow_own]
  Selector/1 -> [omega_to_follow_own]
  Selector2/1 -> [v_to_follow_own]
  Selector1/1 -> Transport Delay/1
  [Qe] -> Matrix Concatenate/4  "Q_s"
  [Pe] -> Matrix Concatenate/2  "P_s"
  Abs/1 -> Matrix Concatenate/3, AVR_Vmeas_Filter/1(in)  "v"
  [omega] -> Matrix Concatenate/1  "omega"
  Cast To Double/1 -> Matrix Concatenate/6
  [connected] -> Memory/1
  Cast To Double1/1 -> Matrix Concatenate/5
  [connect] -> Memory1/1
  [connect] -> connect/3(connect)
  connect/3(connected) -> [connected]
  connect/2(iq_real) -> Matrix Concatenate1/2, trim_output/2(iq), [iq]
  connect/1(id_real) -> Matrix Concatenate1/1, trim_output/1(id), [id]
  Cast To Boolean/1 -> [connect]
  Selector4/1 -> Memory2/1
  Sum8/1 -> Gain1/1, Gain7/1
  [Qe] -> Sum8/1
  Integrator3/1 -> Sum9/2
  Gain7/1 -> Sum9/1
  [Q_s_to_follow_own] -> Sum8/2
  Zero1/1 -> Assignment/1
  Signal Specification/1 -> elec_out/1
  elec_in/1 -> Selector4/1, Selector3/1, Selector2/1, Selector1/1, Selector/1
  Assignment/1 -> Signal Specification/1
  Matrix Concatenate/1 -> Assignment/2
  Matrix Concatenate1/1 -> Signal Specification1/1
  Signal Specification1/1 -> For Each Subsystem/1(In1)
  Constant/1 -> Matrix Concatenate1/3
  For Each Subsystem/1(Out1) -> i/1
  trim_output/1(Out1) -> Terminator2/1
  trim_output/2(Out2) -> Terminator3/1
  trim_output/4(Out4) -> Terminator5/1
  Selector5/1 -> trim_output/3(vd), [vdout]
  Selector6/1 -> [vqout], trim_output/4(vq)
  trim_output/3(Out3) -> Terminator4/1
  v/1 -> Selector6/1, Selector5/1
  Reference frame transform1/1(out_d) -> connect/1(id)
  Reference frame transform1/2(out_q) -> connect/2(iq)
  Gain1/1 -> Integrator3/1
  Memory/1 -> Cast To Double/1
  Memory1/1 -> Cast To Double1/1
  Memory2/1 -> Cast To Boolean/1
  Transport Delay/1 -> [P_s_to_follow_own]
  Reference frame transform2/1(out_d) -> [v_d_PCC]
  Reference frame transform2/2(out_q) -> [v_q_PCC]
  [theta] -> Reference frame transform2/2(theta)
  [vqout] -> Reference frame transform2/3(in_q)
  [vdout] -> Reference frame transform2/1(in_d)
  AVR_Vmeas_Filter/1(out) -> Sum2/2
  Gain4/1 -> Stator circuit/5(vfd)
  Integrator1/1 -> Sum2/1
  [omega_base] -> Selector8/1
  Selector8/1 -> Product4/2
  Product4/1 -> theta/1
  Sum1/1 -> Product4/1
  Selector7/1 -> Sum1/2

== system VFlexP/Grid/Generators/SG ==
  note: Governor
  note: do not rename this block, conditions to initialise the generator from PF result are set on this block's output
  note: port number 1
  note: port number 2
  note: AVR
  elec_in : Inport
  v : Inport  Port=2
  AVR_Exciter : Subsystem  Commented=on  mask{T_s=T_e}
      mask prompts: T_s "Filter time constant"
      mask Display:
      | try
      |     dpoly(1, [T_s, 1])
      | catch
      | end
  AVR_LeadLag : Subsystem  Commented=on  mask{T_2=T_2, T_1=T_1}
      mask help:
      | Transfer function:
      |
      |   1 + sT_2
      | ---------------
      |   1 + sT_1
      mask Display:
      | try
      |     dpoly([T_2, 1], [T_1, 1])
      | catch
      | end
  AVR_MainRegulator : Subsystem  Commented=on  mask{T_s=T_A}
      mask prompts: T_s "Filter time constant"
      mask Display:
      | try
      |     dpoly(1, [T_s, 1])
      | catch
      | end
  AVR_Vmeas_Filter : Subsystem  Commented=on  mask{T_r=0.01}
      mask prompts: T_r "Filter time constant"
      mask Display:
      | try
      |     dpoly(1, [T_r, 1])
      | catch
      | end
  AVR_Vmeas_Filter1 : Subsystem  Commented=through  mask{T_r=0.01}
      mask prompts: T_r "Filter time constant"
      mask Display:
      | try
      |     dpoly(1, [T_r, 1])
      | catch
      | end
  AVR_Vmeas_Filter2 : Subsystem  Commented=through  mask{T_r=0.01}
      mask prompts: T_r "Filter time constant"
      mask Display:
      | try
      |     dpoly(1, [T_r, 1])
      | catch
      | end
  Abs : Abs  Commented=on  SaturateOnIntegerOverflow=off
  Assignment : Assignment  NumberOfDimensions=2  DiagnosticForDimensions=Warning  IndexOptions=Assign all,Index vector (dialog)  Indices=1,block_idx  OutputSizes=1,1
  Cast To Boolean : DataTypeConversion  OutDataTypeStr=boolean  SaturateOnIntegerOverflow=off  RndMeth=Floor
  Cast To Double : DataTypeConversion  OutDataTypeStr=double  SaturateOnIntegerOverflow=off  RndMeth=Floor
  Cast To Double1 : DataTypeConversion  OutDataTypeStr=double  SaturateOnIntegerOverflow=off  RndMeth=Floor
  Complex to Magnitude-Angle1 : ComplexToMagnitudeAngle  Output=Magnitude
  Complex to Magnitude-Angle2 : ComplexToMagnitudeAngle  Output=Magnitude
  Constant : Constant  Value=zeros(1, length(block_buses))  VectorParams1D=off
  Divide : Product  Inputs=*/
  Electromagnetic : Subsystem  Variant=on  VariantControlMode=label  LabelModeActiveChoice=order 2
  For Each Subsystem : Subsystem  TreatAsAtomicUnit=on
  From14 : From  Commented=on  GotoTag=P_s_to_follow_own
  From19 : From  Commented=on  GotoTag=v_d_PCC
  From21 : From  Commented=on  GotoTag=v_q_PCC
  From5 : From  Commented=on  GotoTag=Q_s_to_follow_own
  From6 : From  Commented=on  GotoTag=Q_s
  From7 : From  Commented=on  GotoTag=P_s
  Gain : Gain  Gain=1./R_p
  Gain1 : Gain  Commented=on  Gain=3.4e-4*100
  Gain10 : Gain  Gain=Ps_lf(block_idx)
  Gain2 : Gain  Gain=-1
  Gain3 : Gain  Gain=Sb./gen_static_params.mBase(block_idx)
  Gain4 : Gain  Commented=on  Gain=0
  Gain5 : Gain  Commented=on  Gain=0.01
  Gain6 : Gain  Commented=on  Gain=K_A
  Gain7 : Gain  Commented=on  Gain=0
  Gain8 : Gain  Commented=on  Gain=0
  Integrator : Integrator  Commented=on  InitialCondition=Grid_op_SG.op.States(1).x'
  Integrator1 : Integrator  Commented=on  InitialCondition=Grid_op_SG.op.States(8).x'
  Integrator2 : Integrator  InitialCondition=Grid_op_SG.op.States(4).x'
  Integrator3 : Integrator  Commented=on  InitialCondition=Grid_op_SG.op.States(2).x'
  Integrator4 : Integrator  InitialCondition=Grid_op_SG.op.States(5).x'
  Integrator5 : Integrator  InitialCondition=Grid_op_SG.op.States(6).x'
  LPF2 : Subsystem  Commented=through  mask{T_s=T_g}
      mask prompts: T_s "Filter time constant"
      mask Display:
      | try
      |     dpoly(1, [T_s, 1])
      | catch
      | end
  LPF4 : Subsystem  Commented=through  mask{T_s=0.01}
      mask prompts: T_s "Filter time constant"
      mask Display:
      | try
      |     dpoly(1, [T_s, 1])
      | catch
      | end
  LPF5 : Subsystem  Commented=through  mask{T_s=0.01}
      mask prompts: T_s "Filter time constant"
      mask Display:
      | try
      |     dpoly(1, [T_s, 1])
      | catch
      | end
  Matrix Concatenate : Concatenate  NumInputs=6  Mode=Multidimensional array
  Matrix Concatenate1 : Concatenate  NumInputs=3  Mode=Multidimensional array
  Memory : Memory  InitialCondition=1
  Memory1 : Memory  InitialCondition=1
  Memory2 : Memory  InitialCondition=1
  PIv_d1 : Subsystem  Commented=on
  Product{,1..4} (5 alike) : Product
  Real-Imag to Complex : RealImagToComplex  Commented=on
  Real-Imag to Complex1 : RealImagToComplex
  Real-Imag to Complex2 : RealImagToComplex
  Reference frame transform1 : Subsystem
  Reference frame transform3 : Subsystem
  Rotor axis : Subsystem
  Scope : Scope  Commented=on
      settings: ActiveDisplayYMinimum=3.675  ActiveDisplayYMaximum=3.6927  DataLoggingVariableName=ScopeData2
  Scope1 : Scope
      settings: ActiveDisplayYMinimum=0.95  ActiveDisplayYMaximum=1.05  DataLoggingVariableName=ScopeData3
  Scope2 : Scope  Commented=on
      settings: ActiveDisplayYMinimum=0.24936  ActiveDisplayYMaximum=0.25597
  Scope3 : Scope  NumInputPorts=2
      settings: ActiveDisplayYMinimum=0.29123  ActiveDisplayYMaximum=1.9416  DataLoggingVariableName=ScopeData3
  Selector : Selector  NumberOfDimensions=2  InputPortWidth=3  IndexOptions=Index vector (dialog),Index vector (dialog)  Indices=1,block_idx  OutputSizes=1,1
  Selector1 : Selector  NumberOfDimensions=2  InputPortWidth=3  IndexOptions=Index vector (dialog),Index vector (dialog)  Indices=2,block_idx  OutputSizes=1,1
  Selector2 : Selector  NumberOfDimensions=2  InputPortWidth=3  IndexOptions=Index vector (dialog),Index vector (dialog)  Indices=3,block_idx  OutputSizes=1,1
  Selector3 : Selector  NumberOfDimensions=2  InputPortWidth=3  IndexOptions=Index vector (dialog),Index vector (dialog)  Indices=4,block_idx  OutputSizes=1,1
  Selector4 : Selector  NumberOfDimensions=2  InputPortWidth=3  IndexOptions=Index vector (dialog),Index vector (dialog)  Indices=5,block_idx  OutputSizes=1,1
  Selector5 : Selector  NumberOfDimensions=2  InputPortWidth=3  IndexOptions=Index vector (dialog),Index vector (dialog)  Indices=1,block_buses  OutputSizes=1,1
  Selector6 : Selector  NumberOfDimensions=2  InputPortWidth=3  IndexOptions=Index vector (dialog),Index vector (dialog)  Indices=2,block_buses  OutputSizes=1,1
  Selector7 : Selector  InputPortWidth=length(fref.ref_units)  IndexOptions=Index vector (dialog)  Indices=block_fref  OutputSizes=1
  Selector8 : Selector  InputPortWidth=length(fref.ref_units)  IndexOptions=Index vector (dialog)  Indices=block_fref  OutputSizes=1
  Signal Specification : SignalSpecification  Dimensions=[6 length(buses_lf)]
  Signal Specification1 : SignalSpecification  Dimensions=[3 length(block_buses)]
  Subsystem2 : Subsystem  Commented=through  mask{T_2=-T_W, T_1=0.5*T_W}
      mask help:
      | Transfer function:
      |
      |   1 + sT_2
      | ---------------
      |   1 + sT_1
      mask Display:
      | try
      |     dpoly([T_2, 1], [T_1, 1])
      | catch
      | end
  Subsystem4 : Subsystem  Commented=through  mask{T_2=T_R, T_1=T_R*(R_t/R_p)}
      mask help:
      | Transfer function:
      |
      |   1 + sT_2
      | ---------------
      |   1 + sT_1
      mask Display:
      | try
      |     dpoly([T_2, 1], [T_1, 1])
      | catch
      | end
  Sum1 : Sum  Inputs=|-+
  Sum10 : Sum  Commented=on  Inputs=|+-
  Sum11 : Sum  Commented=on  Inputs=|++
  Sum2 : Sum  Inputs=|+-
  Sum3 : Sum  Inputs=++|
  Sum4 : Sum  Inputs=|-+
  Sum5 : Sum  Inputs=|++
  Sum6 : Sum  Commented=on  Inputs=|-+
  Sum7 : Sum  Commented=on  Inputs=|++
  Sum8 : Sum  Commented=on  Inputs=|-+
  Sum9 : Sum  Commented=on  Inputs=|++
  Terminator{2..5} (4 alike) : Terminator
  Torque : Subsystem
      settings: PortSchema="{\"entries\":[{\"content\":{\"sides\":[{\"content\":{\"connectorIds\":[\"In1\"]},\"type\":\"ConnectorPlacement.EquallySpacedRectSide\",\"uuid\":\"b7abd3bc-22dd-4669-aa40-98bc76884565\"},{\"content\":{\"connectorIds\":[\"In2\",\"In3\",\"Out1\"],\"side\":\"RIGHT\"},\"type\":\"ConnectorPlacement.EquallySpacedRectSide\",\"uuid\":\"e9abb552-b46d-48ed-aa1f-0e9dac604fea\"},{\"content\":{\"connectorIds\":[],\"side\":\"TOP\"},\"type\":\"ConnectorPlacement.EquallySpacedRectSide\",\"uuid\":\"4b14997d-8f32-4cfb-8a1b-18cffb093d28\"}]},\"type\":\"ConnectorPlacement.EquallySpacedConnector\",\"uuid\":\"d6624493-e930-4f0d-8cbe-17f96cb72edc\"}],\"packageUris\":[\"http://schema.mathworks.com/mf0/Connector/R2020b\"],\"version\":\"1.0\"}"
  Zero1 : Constant  Value=zeros(6, length(buses_lf))  VectorParams1D=off  OutDataTypeStr=Inherit: Inherit via back propagation
  connect : Subsystem
  theta : Integrator  InitialCondition=Grid_op_SG.op.States(8).x'  UpperSaturationLimit=2*pi  LowerSaturationLimit=0
  trim_output : Subsystem
  elec_out : Outport
  i : Outport  Port=2
  wires:
  LPF5/1(out) -> [Q_s]
  Reference frame transform1/2(out_q) -> connect/2(iq)
  Product/1 -> Sum4/1
  Product1/1 -> Sum4/2
  theta/1 -> [theta]
  Gain2/1 -> Reference frame transform1/2(theta)
  [theta] -> Reference frame transform3/2(theta)
  Subsystem2/1(Out1) -> Divide/1
  [theta] -> Gain2/1
  LPF2/1(out) -> Subsystem2/1(In1)
  Sum4/1 -> LPF5/1(in)
  Sum5/1 -> LPF4/1(in)
  Product3/1 -> Sum5/2
  [omega_ref] -> Selector7/1  "ref_omega"
  From7/1 -> Sum6/1
  Gain/1 -> Sum3/2
  Product2/1 -> Sum5/1
  Reference frame transform1/1(out_d) -> connect/1(id)
  Sum6/1 -> Gain4/1, Gain5/1
  Integrator/1 -> Sum7/2
  Gain4/1 -> Sum7/1
  Gain5/1 -> Integrator/1
  Subsystem4/1(Out1) -> LPF2/1(in)
  LPF4/1(out) -> [P_s]
  Integrator2/1 -> Sum2/1
  Rotor axis/1(wr) -> Electromagnetic/4(ws), [omega], Scope1/1, Sum1/1, Divide/2, AVR_Vmeas_Filter1/1(in)
  [P_s] -> Matrix Concatenate/2  "P_s"
  [omega] -> Matrix Concatenate/1  "omega"
  Complex to Magnitude-Angle1/1 -> AVR_Vmeas_Filter2/1(in)  "v"
  [Q_s] -> Matrix Concatenate/4  "Q_s"
  Selector3/1 -> [Q_s_to_follow_own]
  Selector/1 -> [omega_to_follow_own]
  Selector1/1 -> Gain10/1
  Selector2/1 -> [v_to_follow_own]
  [connect] -> Memory1/1
  [connected] -> Memory/1
  Cast To Double1/1 -> Matrix Concatenate/5
  Cast To Double/1 -> Matrix Concatenate/6
  From14/1 -> Sum6/2
  Real-Imag to Complex1/1 -> Complex to Magnitude-Angle1/1
  [vdout] -> Product/1, Product2/1
  [vqout] -> Product3/1, Product1/2
  [v_d_PCC] -> Real-Imag to Complex1/1  "vod"
  [v_q_PCC] -> Real-Imag to Complex1/2  "voq"
  Sum7/1 -> Sum3/1
  connect/3(connected) -> [connected]
  [connect] -> connect/3(connect)
  connect/1(id_real) -> Real-Imag to Complex2/1, trim_output/1(id), Matrix Concatenate1/1, Product1/1, Product2/2
  Selector4/1 -> Cast To Boolean/1
  Cast To Boolean/1 -> Memory2/1
  From5/1 -> Sum8/2
  Gain8/1 -> Integrator3/1
  Gain7/1 -> Sum9/1
  Integrator3/1 -> Sum9/2
  Sum8/1 -> Gain8/1, Gain7/1
  From6/1 -> Sum8/1
  Zero1/1 -> Assignment/1
  Signal Specification/1 -> elec_out/1
  elec_in/1 -> Selector4/1, Selector3/1, Selector2/1, Selector1/1, Selector/1
  Assignment/1 -> Signal Specification/1
  Matrix Concatenate/1 -> Assignment/2
  Matrix Concatenate1/1 -> Signal Specification1/1
  Signal Specification1/1 -> For Each Subsystem/1(In1)
  Constant/1 -> Matrix Concatenate1/3
  For Each Subsystem/1(Out1) -> i/1
  connect/2(iq_real) -> Product3/2, Product/2, Real-Imag to Complex2/2, trim_output/2(iq), Matrix Concatenate1/2
  trim_output/3(Out3) -> Terminator4/1
  trim_output/1(Out1) -> Terminator2/1
  trim_output/4(Out4) -> Terminator5/1
  trim_output/2(Out2) -> Terminator3/1
  v/1 -> Selector6/1, Selector5/1
  Selector5/1 -> [vdout], trim_output/3(vd)
  Selector6/1 -> [vqout], trim_output/4(vq)
  [vqout] -> Reference frame transform3/3(in_q)
  [vdout] -> Reference frame transform3/1(in_d)
  Reference frame transform3/1(out_d) -> [v_d_PCC]
  Reference frame transform3/2(out_q) -> [v_q_PCC]
  Memory/1 -> Cast To Double/1
  Gain10/1 -> [P_s_to_follow_own]
  Memory1/1 -> Cast To Double1/1
  Memory2/1 -> [connect]
  Selector7/1 -> Sum1/2
  Selector8/1 -> Product4/2
  [omega_base] -> Selector8/1
  Product4/1 -> theta/1
  Sum1/1 -> Product4/1
  Sum3/1 -> Subsystem4/1(In1)
  Sum2/1 -> Gain/1
  Torque/1(te) -> Gain3/1
  Gain3/1 -> Rotor axis/1(te)
  Integrator1/1 -> Sum10/1
  AVR_MainRegulator/1(out) -> AVR_LeadLag/1(In1)
  AVR_Vmeas_Filter/1(out) -> Sum10/2
  AVR_Exciter/1(out) -> Gain1/1
  AVR_LeadLag/1(Out1) -> AVR_Exciter/1(in)
  From19/1 -> Real-Imag to Complex/1
  Abs/1 -> AVR_Vmeas_Filter/1(in)  "v"
  From21/1 -> Real-Imag to Complex/2
  Real-Imag to Complex/1 -> Abs/1
  Sum11/1 -> AVR_MainRegulator/1(in)
  Gain6/1 -> Sum11/1
  PIv_d1/1(vfd) -> Gain6/1
  Sum10/1 -> Scope/1, PIv_d1/1(In1)
  Gain1/1 -> Scope2/1
  AVR_Vmeas_Filter1/1(out) -> Sum2/2
  AVR_Vmeas_Filter2/1(out) -> Matrix Concatenate/3, Scope3/1
  Integrator5/1 -> Rotor axis/2(tm)
  Real-Imag to Complex2/1 -> Complex to Magnitude-Angle2/1
  Complex to Magnitude-Angle2/1 -> Scope3/2  "v"
  Electromagnetic/2(isq) -> [isq], Torque/3(isq), Reference frame transform1/3(in_q)
  Electromagnetic/1(isd) -> Reference frame transform1/1(in_d), Torque/2(isd), [isd]
  [v_d_PCC] -> Electromagnetic/1(vsd)
  [v_q_PCC] -> Electromagnetic/2(vsq)
  Integrator4/1 -> Electromagnetic/3(vfd)
  Electromagnetic/3(psi) -> Torque/1(psi)
